simulink model "SolarPannal_Simulink"  (R2023a)
settings: Solver=VariableStepAuto  StartTime=0.0  StopTime=54000  RelTol=1e-3
model workspace (MAT data in the model file):
  J = 8.6
  Kd = 5
  Kf = 0.07
  Kg = 2000
  Kt = 0.07
  L = 1e-05
  R = 10
libraries: slpidlib x1
settings Model: Creator=hyyxl  LastModifiedBy=hyyxl
settings DataIOCC: ExternalInput=[sunTime, sunPosition]  LoadExternalInput=on

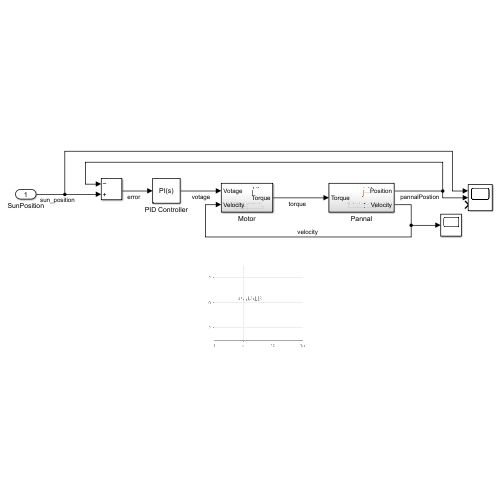
[thumbnail: Simulink's stored preview of the top-level diagram]
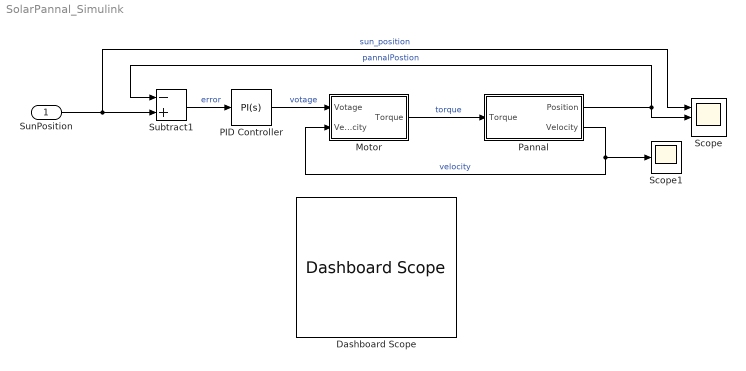
== system SolarPannal_Simulink ==
  SunPosition : Inport
  Dashboard Scope : DashboardScope
  Motor : Subsystem
  PID Controller : slpidlib/PID Controller  Controller=PI  Form=Parallel  TimeDomain=Continuous-time  UseExternalTs=off  SampleTime=-1  IntegratorMethod=Forward Euler  FilterMethod=Forward Euler  ControllerParametersSource=internal  P=200  I=150  UseKiTs=off  D=0  N=100  UseFilter=on  TunerSelectOption=Transfer Function Based (PID Tuner App)  InitialConditionSource=internal  InitialConditionForIntegrator=0  InitialConditionForFilter=0  DifferentiatorICPrevScaledInput=0  ExternalReset=none  TrackingMode=off  Kt=1  LimitOutput=off  SatLimitsSource=internal  UpperSaturationLimit=inf  LowerSaturationLimit=-inf  LinearizeAsGain=on  AntiWindupMode=none  Kb=1  LimitIntegrator=off  UpperIntegratorSaturationLimit=inf  LowerIntegratorSaturationLimit=-inf  POutMin=[]  POutMax=[]  IOutMin=[]  IOutMax=[]  DOutMin=[]  DOutMax=[]  NOutMin=[]  NOutMax=[]  SumOutMin=[]  SumOutMax=[]  SaturationOutMin=[]  SaturationOutMax=[]  PParamMin=[]  PParamMax=[]  IParamMin=[]  IParamMax=[]  DParamMin=[]  DParamMax=[]  NParamMin=[]  NParamMax=[]  KbParamMin=[]  KbParamMax=[]  KtParamMin=[]  KtParamMax=[]  KbOutMin=[]  KbOutMax=[]  KtOutMin=[]  KtOutMax=[]  IntegratorOutMin=[]  IntegratorOutMax=[]  FilterOutMin=[]  FilterOutMax=[]  SumI1OutMin=[]  SumI1OutMax=[]  SumI2OutMin=[]  SumI2OutMax=[]  SumI3OutMin=[]  SumI3OutMax=[]  SumI4OutMin=[]  SumI4OutMax=[]  SumDOutMin=[]  SumDOutMax=[]  DifferentiatorOutMin=[]  DifferentiatorOutMax=[]  FilterDiffOutCoefMin=[]  FilterDiffOutCoefMax=[]  ReciprocalOutMin=[]  ReciprocalOutMax=[]  SumDenOutMin=[]  SumDenOutMax=[]  SumNumOutMin=[]  SumNumOutMax=[]  DivideOutMin=[]  DivideOutMax=[]  UdiffTsProdOutMin=[]  UdiffTsProdOutMax=[]  NTsProdOutMin=[]  NTsProdOutMax=[]  UintegralTsProdOutMin=[]  UintegralTsProdOutMax=[]  UngainTsProdOutMin=[]  UngainTsProdOutMax=[]  ClampingZeroOutDataTypeStr=Inherit: Inherit via back propagation  ClampingZeroOutMin=[]  ClampingZeroOutMax=[]  FilterDenConstantOutDataTypeStr=Inherit: Inherit via back propagation  FilterDenConstantOutMin=[]  FilterDenConstantOutMax=[]  PCopyOutDataTypeStr=Inherit: Inherit via back propagation  PCopyOutMin=[]  PCopyOutMax=[]  NCopyOutDataTypeStr=Inherit: Inherit via back propagation  NCopyOutMin=[]  NCopyOutMax=[]  IntegratorContinuousStateAttributes=''  IntegratorStateMustResolveToSignalObject=off  IntegratorRTWStateStorageClass=Auto  FilterContinuousStateAttributes=''  FilterStateMustResolveToSignalObject=off  FilterRTWStateStorageClass=Auto  ParallelPVariant=InternalParameters  IdealPVariant=Disabled  IVariant=InternalParameters  DVariant=Disabled  IntegratorVariant=Continuous  SatVariant=Disabled  AWVariant=Passthrough  PCopyVariant=Disabled  TRVariant=Disabled  FdbkBlocksVariant=Forward  IdealPFdbkVariant=Disabled  SatFdbkVariant=Disabled  DerivativeFilterVariant=Disabled  NVariant=Disabled  NCopyVariant=Disabled_SignalSpec  FilterICVariant=Disabled  IntegratorICVariant=InternalICs  ExternalResetVariant=Disabled  TRSumVariant=Passthrough  SumFdbkVariant=Disabled  SumVariant=Sum_PI  TsampFilterVariant=InternalTs  TsampNgainVariant=Passthrough  TsampIntegralVariant=Disabled_SignalSpec  ExternalSaturationOutDataTypeStr=Inherit: Same as second input
  Pannal : Subsystem
  Scope : Scope  NumInputPorts=3
  Scope1 : Scope
  Subtract1 : Sum  Inputs=-+
  wires:
  Pannal/2(Velocity) -> Motor/2(Velocity), Scope1/1  "velocity"
  SunPosition/1 -> Subtract1/2, Scope/1  "sun_position"
  Motor/1(Torque) -> Pannal/1(Torque)  "torque"
  Pannal/1(Position) -> Subtract1/1, Scope/2  "pannalPostion"
  PID Controller/1 -> Motor/1(Votage)  "votage"
  Subtract1/1 -> PID Controller/1  "error"

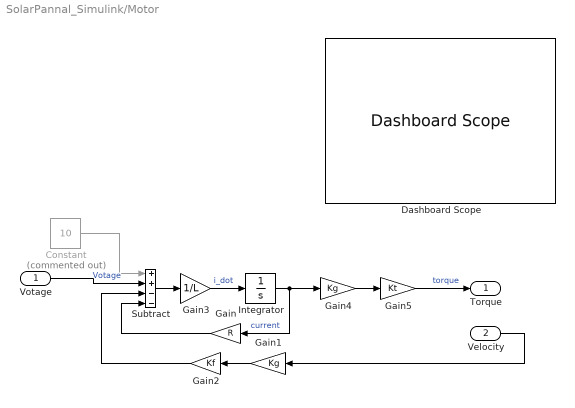
== system SolarPannal_Simulink/Motor ==
  Votage : Inport
  Velocity : Inport  Port=2
  Constant : Constant  Commented=on  Value=10
  Dashboard Scope : DashboardScope
  Gain : Gain  Gain=R
  Gain1 : Gain  Gain=Kg
  Gain2 : Gain  Gain=Kf
  Gain3 : Gain  Gain=1/L
  Gain4 : Gain  Gain=Kg
  Gain5 : Gain  Gain=Kt
  Integrator : Integrator
  Subtract : Sum  Inputs=++--
  Torque : Outport
  wires:
  Gain4/1 -> Gain5/1
  Gain1/1 -> Gain2/1
  Gain/1 -> Subtract/4
  Integrator/1 -> Gain/1, Gain4/1  "current"
  Gain3/1 -> Integrator/1  "i_dot"
  Gain5/1 -> Torque/1  "torque"
  Gain2/1 -> Subtract/3
  Subtract/1 -> Gain3/1
  Votage/1 -> Subtract/2  "Votage"
  Velocity/1 -> Gain1/1
  Constant/1 -> Subtract/1

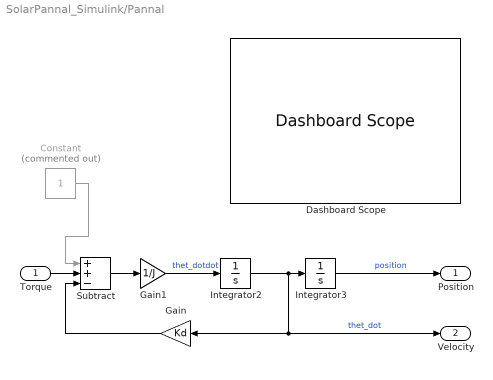
== system SolarPannal_Simulink/Pannal ==
  Torque : Inport
  Constant : Constant  Commented=on
  Dashboard Scope : DashboardScope
  Gain : Gain  Gain=Kd
  Gain1 : Gain  Gain=1/J
  Integrator2 : Integrator
  Integrator3 : Integrator
  Subtract : Sum  Inputs=++-
  Position : Outport
  Velocity : Outport  Port=2
  wires:
  Integrator3/1 -> Position/1  "position"
  Integrator2/1 -> Velocity/1, Gain/1, Integrator3/1  "thet_dot"
  Gain1/1 -> Integrator2/1  "thet_dotdot"
  Gain/1 -> Subtract/3
  Subtract/1 -> Gain1/1
  Torque/1 -> Subtract/2
  Constant/1 -> Subtract/1
